simulink model "processus_kalman"  (R2023b)
settings: Solver=ode45  StartTime=0.0  StopTime=10.0  FixedStep=0.0001  MaxStep=0.001  RelTol=1e-4  EnableMultiTasking=on
values from neighbouring files (symbols this model uses):
  Km = 0.0281    [simu.m]
  Kv = -identified_model.A(2,2)    [id_RT_ar.m]    (also in simu.m = 1.772e-05)
  m = 7.4e-5    (= 7.4e-05)    [cost_iae_n.m]    (also in main_ga_n.m; simu.m)
  P0 = [1e-17 0 0;0 1e-17 0;0 0 3e-20]    [simu.m]
  Q = real(Q)    [calcul_Q.m]    (also in simu.m = calcul_Q(Km,Kv,m,Te,W))
  R = (3e-8)^2    (= 9e-16)    [config_kalman.m]    (also in reglage_filtre_kalman.m; simu.m = 1e-16)
  Te = 0.001    [simu.m]
  X0 = [0 0 0]'    [simu.m]
undefined symbols (not defined in the file or in its folder): A_disc, C_disc
settings Model: Creator=emmanuel.piat  LastModifiedBy=ekole
settings SolverCC: InitialStep=0.0001  AlgebraicLoopSolver=TrustRegion
settings DataIOCC: SaveFormat=Array  SignalLoggingSaveFormat=ModelDataLogs  ReturnWorkspaceOutputs=off
settings OptimizationCC: BlockReduction=off  BooleanDataType=off  ExpressionDepthLimit=2147483647  InitFltsAndDblsToZero=on  LifeSpan=inf
settings DebuggingCC: SaveWithParameterizedLinksMsg=none  UnderspecifiedInitializationDetection=Classic  MergeDetectMultiDrivingBlocksExec=none  SignalResolutionControl=TryResolveAllWithWarning  MultiTaskDSMMsg=warning  MultiTaskCondExecSysMsg=none  FcnCallInpInsideContextMsg=warning  UnconnectedInputMsg=warning  UnconnectedOutputMsg=warning  UnconnectedLineMsg=warning  StateNameClashWarn=warning  SFUnexpectedBacktrackingDiag=warning  SFNoUnconditionalDefaultTransitionDiag=warning  SFExecutionAtInitializationDiag=none  ArithmeticOperatorsInVariantConditions=warning
settings HardwareCC: ProdBitPerPointer=32  ProdBitPerSizeT=32  ProdBitPerPtrDiffT=32  ProdLargestAtomicFloat=None  ProdIntDivRoundTo=Undefined  ProdEndianess=Unspecified  ProdWordSize=32  ProdHWDeviceType=32-bit Generic  TargetUnknown=on
settings ModelReferenceCC: PropagateSignalLabelsOutOfModel=off
settings CodeAppCC: StateflowObjectComments=on
settings GRTTargetCC: TargetLangStandard=C89/C90 (ANSI)  ModelReferenceCompliant=off  CompOptLevelCompliant=off  CombineOutputUpdateFcns=off  MatFileLogging=off  GRTInterface=on
settings ConfigComp: CovMetricSettings=dw  CovSaveCumulativeToWorkspaceVar=on  CovSaveSingleToWorkspaceVar=on

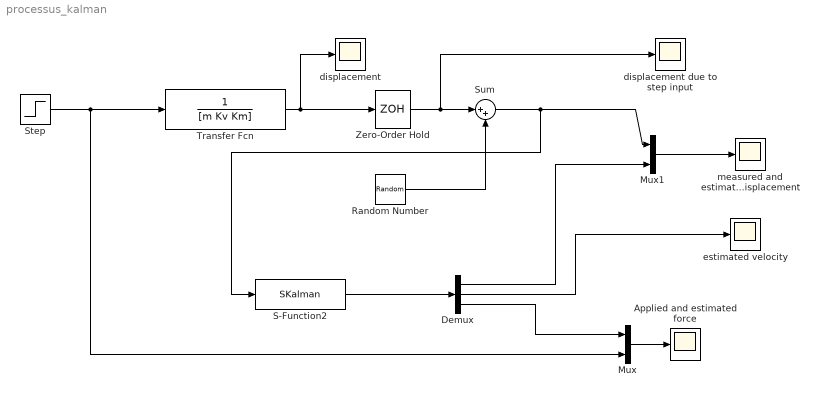
== system processus_kalman ==
  Applied and estimated force : Scope
  Demux : Demux  Outputs=3
      settings: DisplayOption=none
  Mux : Mux  Inputs=2
  Mux1 : Mux  Inputs=2
  Random Number : RandomNumber  Variance=R  SampleTime=Te
  S-Function2 : S-Function  FunctionName=SKalman  Parameters=A_disc,C_disc,Q,R,X0,P0,Te  SFunctionDeploymentMode=off  EnableBusSupport=off
  Step : Step  After=10e-9  SampleTime=0
  Sum : Sum  Inputs=|++  InputSameDT=on  SaturateOnIntegerOverflow=on  OutDataTypeStr=Inherit: Same as first input
  Transfer Fcn : TransferFcn  Denominator=[m Kv Km]
  Zero-Order Hold : ZeroOrderHold  SampleTime=Te
  displacement : Scope
  "displacement due to step input " : Scope
  estimated velocity : Scope
  measured and estimated displacement : Scope
  wires:
  Random Number/1 -> Sum/2
  Zero-Order Hold/1 -> Sum/1, "displacement due to step input "/1
  Transfer Fcn/1 -> Zero-Order Hold/1, displacement/1
  Sum/1 -> S-Function2/1, Mux1/1
  Mux/1 -> Applied and estimated force/1
  Demux/3 -> Mux/1
  Demux/2 -> estimated velocity/1
  Mux1/1 -> measured and estimated displacement/1
  Demux/1 -> Mux1/2
  Step/1 -> Transfer Fcn/1, Mux/2
  S-Function2/1 -> Demux/1
